simulink model "sampleIT"  (R2018a)
settings: Solver=FixedStepDiscrete  StartTime=0.0  StopTime=10.0  FixedStep=.001  RelTol=1e-3
libraries: simulink x1
settings Model: Creator=mattclark  LastModifiedBy=mattclark
settings SFSimCC: SimCustomHeaderCode=|
  | #include "sampleIT.h"
  | #include "monitor.h"
settings SFSimCC: SimUserSources=|
  | sampleIT.c
  | monitor.c

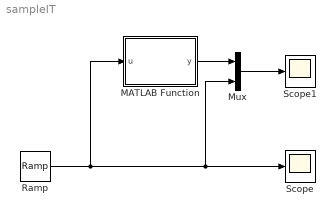
== system sampleIT ==
  MATLAB Function : MATLAB Function  TreatAsAtomicUnit=on
  Mux : Mux  Inputs=2
  Ramp : simulink/Sources/Ramp  slope=1  start=0  InitialOutput=0
  Scope : Scope
  Scope1 : Scope
  wires:
  Ramp/1 -> MATLAB Function/1(u), Mux/2, Scope/1
  MATLAB Function/1(y) -> Mux/1
  Mux/1 -> Scope1/1

== matlab function sampleIT/MATLAB Function ==
  data: u input; y output
function y = sampleIT(u)
y = 0.0;
y = coder.ceval('sampleIT',u);
